simulink model "timedIzhikevichTest"  (R2020a)
settings: Solver=FixedStepAuto  StartTime=0.0  StopTime=12  FixedStep=0.001  RelTol=1e-3
libraries: simulink x2, dspsigops x1
settings Model: Creator=40129232  LastModifiedBy=40175607
settings DataIOCC: ReturnWorkspaceOutputs=off
settings OptimizationCC: LifeSpan=inf
settings DebuggingCC: SFExecutionAtInitializationDiag=none  ArithmeticOperatorsInVariantConditions=warning
settings SFSimCC: SimUseLocalCustomCode=off  CustomCodeUndefinedFunction=UseInterfaceOnly
settings RTWCC: RTWUseLocalCustomCode=off
settings CodeAppCC: StateflowObjectComments=on

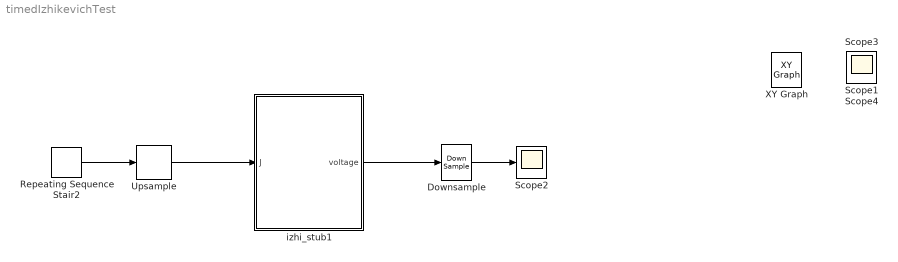
== system timedIzhikevichTest ==
  Downsample : DownSample  N=12  RateOptions=Allow multirate processing
  Repeating Sequence Stair2 : simulink/Sources/Repeating Sequence Stair  OutValues=[40.37, 52.35, 62.17, 70.19, 76.75].'  tsamp=0.012  OutMin=[]  OutMax=[]  OutDataTypeStr=double  OutputDataTypeScalingMode=double  OutDataType=fixdt(0,8)  ConRadixGroup=Best Precision: Vector-wise  OutScaling=2^-12
  Scope{1..4} (4 alike) : Scope
  Upsample : dspsigops/Upsample  N=12  phase=0  RateOptions=Allow multirate processing  ic=0  mode=Unused parameter value
  izhi_stub1 : Subsystem
  XY Graph : simulink/Sinks/XY Graph  IOType=viewer  xmin=-1  xmax=1  ymin=-1  ymax=1  st=-1
  wires:
  Repeating Sequence Stair2/1 -> Upsample/1
  izhi_stub1/1(voltage) -> Downsample/1
  Downsample/1 -> Scope2/1
  Upsample/1 -> izhi_stub1/1(J)

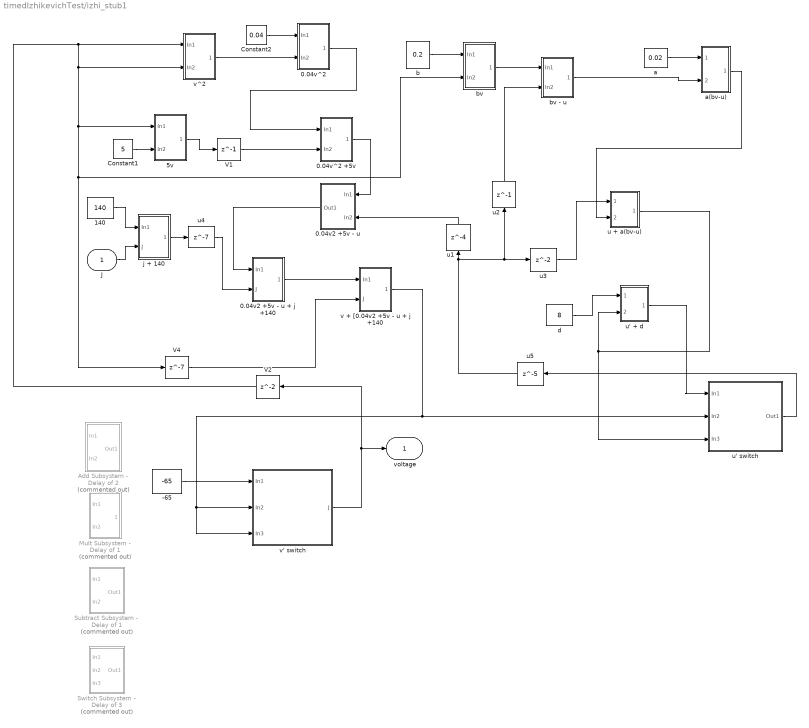
== system timedIzhikevichTest/izhi_stub1 ==
  J : Inport
  -65 : Constant  Value=-65
  0.04v2 +5v - u : Subsystem
  0.04v2 +5v - u + j +140 : Subsystem
  0.04v^2 : Subsystem
  0.04v^2 +5v : Subsystem
  140 : Constant  Value=140
  5v : Subsystem
  Add Subsystem - Delay of 2 : Subsystem  Commented=on
  Constant1 : Constant  Value=5
  Constant2 : Constant  Value=0.04
  Mult Subsystem - Delay of 1 : Subsystem  Commented=on
  Subtract Subsystem - Delay of 1 : Subsystem  Commented=on
  Switch Subsystem - Delay of 3 : Subsystem  Commented=on
  V1 : Delay  DelayLength=1  InitialCondition=0
  V2 : Delay  InitialCondition=0
  V4 : Delay  DelayLength=7  InitialCondition=0
  a : Constant  Value=0.02
  a(bv-u) : Subsystem
  b : Constant  Value=0.2
  bv : Subsystem
  bv - u : Subsystem
  d : Constant  Value=8
  j + 140 : Subsystem
  u + a(bv-u) : Subsystem
  u' + d : Subsystem
  u' switch : Subsystem
  u1 : Delay  DelayLength=4  InitialCondition=0
  u2 : Delay  DelayLength=1  InitialCondition=0
  u3 : Delay  InitialCondition=0
  u4 : Delay  DelayLength=7  InitialCondition=0
  u5 : Delay  DelayLength=5  InitialCondition=0
  v + [0.04v2 +5v - u + j +140 : Subsystem
  v' switch : Subsystem
  v^2 : Subsystem
  voltage : Outport  VectorParamsAs1DForOutWhenUnconnected=off
  wires:
  d/1 -> u' + d/1(In1)
  Constant1/1 -> 5v/2(In2)
  Constant2/1 -> 0.04v^2/1(In1)
  140/1 -> j + 140/1(In1)
  -65/1 -> v' switch/1(In1)
  b/1 -> bv/1(In1)
  a/1 -> a(bv-u)/1(In1)
  5v/1(Out1) -> V1/1
  v' switch/1(J) -> V2/1, voltage/1
  v^2/1(Out1) -> 0.04v^2/2(In2)
  V1/1 -> 0.04v^2 +5v/2(In2)
  bv/1(Out1) -> bv - u/1(In1)
  0.04v^2/1(Out1) -> 0.04v^2 +5v/1(In1)
  0.04v^2 +5v/1(Out1) -> 0.04v2 +5v - u/1(In1)
  u1/1 -> 0.04v2 +5v - u/2(In2)
  u2/1 -> bv - u/2(In2)
  u' switch/1(Out1) -> u5/1
  u3/1 -> u + a(bv-u)/1(In1)
  bv - u/1(Out1) -> a(bv-u)/2(In2)
  a(bv-u)/1(Out1) -> u + a(bv-u)/2(In2)
  j + 140/1(Out1) -> u4/1
  0.04v2 +5v - u/1(Out1) -> 0.04v2 +5v - u + j +140/1(In1)
  J/1 -> j + 140/2(J)
  V4/1 -> v + [0.04v2 +5v - u + j +140/2(J)
  u4/1 -> 0.04v2 +5v - u + j +140/2(J)
  0.04v2 +5v - u + j +140/1(Out1) -> v + [0.04v2 +5v - u + j +140/1(In1)
  u' + d/1(Out1) -> u' switch/1(In1)
  u + a(bv-u)/1(Out1) -> u' switch/3(In3), u' + d/2(In2)
  u5/1 -> u3/1, u2/1, u1/1
  v + [0.04v2 +5v - u + j +140/1(Out1) -> u' switch/2(In2), v' switch/3(In3), v' switch/2(In2)
  V2/1 -> v^2/1(In1), v^2/2(In2), 5v/1(In1), V4/1, bv/2(In2)

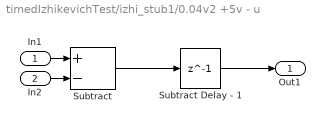
== system timedIzhikevichTest/izhi_stub1/0.04v2 +5v - u ==
  In1 : Inport
  In2 : Inport  Port=2
  Subtract : Sum  Inputs=+-
  Subtract Delay - 1 : Delay  DelayLength=1
  Out1 : Outport
  wires:
  In1/1 -> Subtract/1
  Subtract/1 -> Subtract Delay - 1/1
  Subtract Delay - 1/1 -> Out1/1
  In2/1 -> Subtract/2

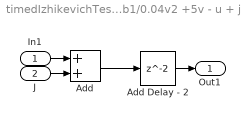
== system timedIzhikevichTest/izhi_stub1/0.04v2 +5v - u + j +140 ==
  In1 : Inport
  J : Inport  Port=2
  Add : Sum
  Add Delay - 2 : Delay
  Out1 : Outport
  wires:
  Add Delay - 2/1 -> Out1/1
  Add/1 -> Add Delay - 2/1
  In1/1 -> Add/1
  J/1 -> Add/2

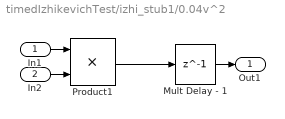
== system timedIzhikevichTest/izhi_stub1/0.04v^2 ==
  In1 : Inport
  In2 : Inport  Port=2
  Mult Delay - 1 : Delay  DelayLength=1
  Product1 : Product
  Out1 : Outport
  wires:
  Product1/1 -> Mult Delay - 1/1
  Mult Delay - 1/1 -> Out1/1
  In2/1 -> Product1/2
  In1/1 -> Product1/1

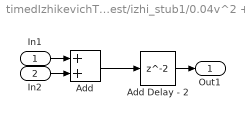
== system timedIzhikevichTest/izhi_stub1/0.04v^2 +5v ==
  In1 : Inport
  In2 : Inport  Port=2
  Add : Sum
  Add Delay - 2 : Delay
  Out1 : Outport
  wires:
  Add Delay - 2/1 -> Out1/1
  Add/1 -> Add Delay - 2/1
  In1/1 -> Add/1
  In2/1 -> Add/2

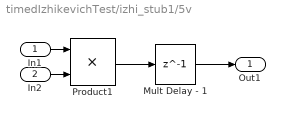
== system timedIzhikevichTest/izhi_stub1/5v ==
  In1 : Inport
  In2 : Inport  Port=2
  Mult Delay - 1 : Delay  DelayLength=1
  Product1 : Product
  Out1 : Outport
  wires:
  Product1/1 -> Mult Delay - 1/1
  Mult Delay - 1/1 -> Out1/1
  In2/1 -> Product1/2
  In1/1 -> Product1/1

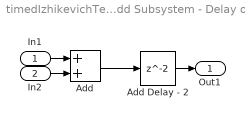
== system timedIzhikevichTest/izhi_stub1/Add Subsystem - Delay of 2 ==
  In1 : Inport
  In2 : Inport  Port=2
  Add : Sum
  Add Delay - 2 : Delay
  Out1 : Outport
  wires:
  Add Delay - 2/1 -> Out1/1
  Add/1 -> Add Delay - 2/1
  In1/1 -> Add/1
  In2/1 -> Add/2

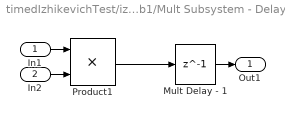
== system timedIzhikevichTest/izhi_stub1/Mult Subsystem - Delay of 1 ==
  In1 : Inport
  In2 : Inport  Port=2
  Mult Delay - 1 : Delay  DelayLength=1
  Product1 : Product
  Out1 : Outport
  wires:
  Product1/1 -> Mult Delay - 1/1
  Mult Delay - 1/1 -> Out1/1
  In2/1 -> Product1/2
  In1/1 -> Product1/1

== system timedIzhikevichTest/izhi_stub1/Subtract Subsystem - Delay of 1 ==
  In1 : Inport
  In2 : Inport  Port=2
  Subtract : Sum  Inputs=+-
  Subtract Delay - 1 : Delay  DelayLength=1
  Out1 : Outport
  wires:
  In1/1 -> Subtract/1
  Subtract/1 -> Subtract Delay - 1/1
  Subtract Delay - 1/1 -> Out1/1
  In2/1 -> Subtract/2

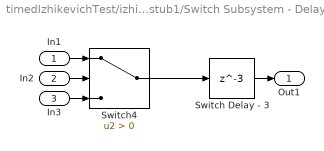
== system timedIzhikevichTest/izhi_stub1/Switch Subsystem - Delay of 3 ==
  In1 : Inport
  In2 : Inport  Port=2
  In3 : Inport  Port=3
  Switch Delay - 3 : Delay  DelayLength=3
  Switch4 : Switch  Criteria=u2 > Threshold
  Out1 : Outport
  wires:
  In2/1 -> Switch4/2
  Switch4/1 -> Switch Delay - 3/1
  In1/1 -> Switch4/1
  Switch Delay - 3/1 -> Out1/1
  In3/1 -> Switch4/3

== system timedIzhikevichTest/izhi_stub1/a(bv-u) ==
  In1 : Inport
  In2 : Inport  Port=2
  Mult Delay - 1 : Delay  DelayLength=1
  Product1 : Product
  Out1 : Outport
  wires:
  Product1/1 -> Mult Delay - 1/1
  Mult Delay - 1/1 -> Out1/1
  In2/1 -> Product1/2
  In1/1 -> Product1/1

== system timedIzhikevichTest/izhi_stub1/bv ==
  In1 : Inport
  In2 : Inport  Port=2
  Mult Delay - 1 : Delay  DelayLength=1
  Product1 : Product
  Out1 : Outport
  wires:
  Product1/1 -> Mult Delay - 1/1
  Mult Delay - 1/1 -> Out1/1
  In2/1 -> Product1/2
  In1/1 -> Product1/1

== system timedIzhikevichTest/izhi_stub1/bv - u ==
  In1 : Inport
  In2 : Inport  Port=2
  Subtract : Sum  Inputs=+-
  Subtract Delay - 1 : Delay  DelayLength=1
  Out1 : Outport
  wires:
  In1/1 -> Subtract/1
  Subtract/1 -> Subtract Delay - 1/1
  Subtract Delay - 1/1 -> Out1/1
  In2/1 -> Subtract/2

== system timedIzhikevichTest/izhi_stub1/j + 140 ==
  In1 : Inport
  J : Inport  Port=2
  Add : Sum
  Add Delay - 2 : Delay
  Out1 : Outport
  wires:
  Add Delay - 2/1 -> Out1/1
  Add/1 -> Add Delay - 2/1
  In1/1 -> Add/1
  J/1 -> Add/2

== system timedIzhikevichTest/izhi_stub1/u + a(bv-u) ==
  In1 : Inport
  In2 : Inport  Port=2
  Add : Sum
  Add Delay - 2 : Delay
  Out1 : Outport
  wires:
  Add Delay - 2/1 -> Out1/1
  Add/1 -> Add Delay - 2/1
  In1/1 -> Add/1
  In2/1 -> Add/2

== system timedIzhikevichTest/izhi_stub1/u' + d ==
  In1 : Inport
  In2 : Inport  Port=2
  Add : Sum
  Add Delay - 2 : Delay
  Out1 : Outport
  wires:
  Add Delay - 2/1 -> Out1/1
  Add/1 -> Add Delay - 2/1
  In1/1 -> Add/1
  In2/1 -> Add/2

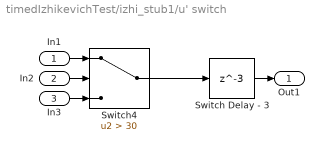
== system timedIzhikevichTest/izhi_stub1/u' switch ==
  In1 : Inport
  In2 : Inport  Port=2
  In3 : Inport  Port=3
  Switch Delay - 3 : Delay  DelayLength=3
  Switch4 : Switch  Criteria=u2 > Threshold  Threshold=30
  Out1 : Outport
  wires:
  In2/1 -> Switch4/2
  Switch4/1 -> Switch Delay - 3/1
  In1/1 -> Switch4/1
  Switch Delay - 3/1 -> Out1/1
  In3/1 -> Switch4/3

== system timedIzhikevichTest/izhi_stub1/v + [0.04v2 +5v - u + j +140 ==
  In1 : Inport
  J : Inport  Port=2
  Add : Sum
  Add Delay - 2 : Delay
  Out1 : Outport
  wires:
  Add Delay - 2/1 -> Out1/1
  Add/1 -> Add Delay - 2/1
  In1/1 -> Add/1
  J/1 -> Add/2

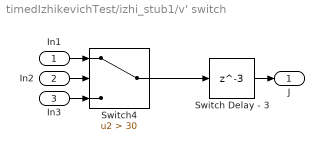
== system timedIzhikevichTest/izhi_stub1/v' switch ==
  In1 : Inport
  In2 : Inport  Port=2
  In3 : Inport  Port=3
  Switch Delay - 3 : Delay  DelayLength=3
  Switch4 : Switch  Criteria=u2 > Threshold  Threshold=30
  J : Outport
  wires:
  In2/1 -> Switch4/2
  Switch4/1 -> Switch Delay - 3/1
  In1/1 -> Switch4/1
  Switch Delay - 3/1 -> J/1
  In3/1 -> Switch4/3

== system timedIzhikevichTest/izhi_stub1/v^2 ==
  In1 : Inport
  In2 : Inport  Port=2
  Mult Delay - 2 : Delay  DelayLength=1
  Product1 : Product
  Out1 : Outport
  wires:
  Product1/1 -> Mult Delay - 2/1
  In2/1 -> Product1/2
  In1/1 -> Product1/1
  Mult Delay - 2/1 -> Out1/1
